simulink model "HipMotor"  (R2016a)
settings: Solver=VariableStepAuto  StartTime=0.0  StopTime=10.0  RelTol=1e-3
settings Model: Creator=MyPC  LastModifiedBy=MyPC

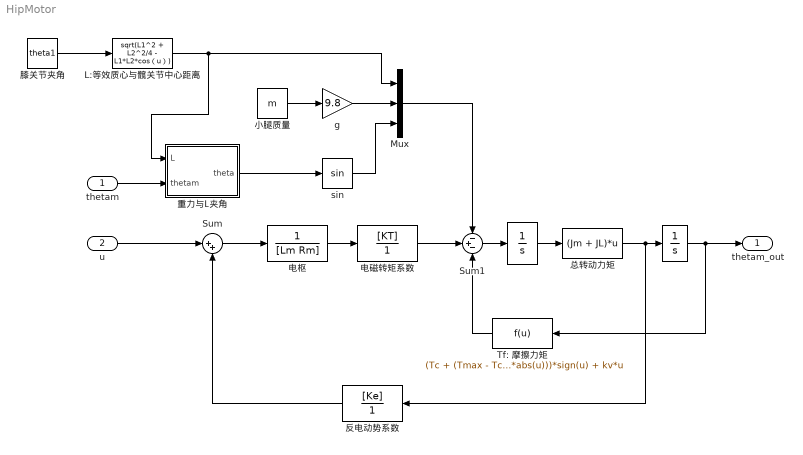
== system HipMotor ==
  thetam : Inport
  u : Inport  Port=2
  " " : TransferFcn  Denominator=[1 0]
  " " : TransferFcn  Denominator=[1 0]
  L:等效质心与髋关节中心距离 : Fcn  Expr=sqrt(L1^2 + L2^2/4 - L1*L2*cos（u）)  mask{L2=0.3, L1=0.3}
  Mux : Mux  Inputs=3
  Sum : Sum  Inputs=|++
  Sum1 : Sum  Inputs=-+-
  Tf: 摩擦力矩 : Fcn  Expr=(Tc + (Tmax - Tc)*exp(-v*abs(u)))*sign(u) + kv*u  mask{Tc=0.05, Tmax=0.06, v=0.01, kv=0.02}
  g : Gain  Gain=9.8
  sin : Trigonometry
  反电动势系数 : TransferFcn  Numerator=[Ke]  Denominator=[1]  mask{Ke=0.444}
  小腿质量 : Constant  Value=m  mask{m=5}
  总转动力矩 : Fcn  Expr=(Jm + JL)*u  mask{Jm=1.39e-4, JL=0.2}
  电枢 : TransferFcn  Denominator=[Lm Rm]  mask{Lm=2.34, Rm=5.48}
  电磁转矩系数 : TransferFcn  Numerator=[KT]  Denominator=[1]  mask{KT=0.443}
  膝关节夹角 : Constant  Value=theta1  mask{theta1=1.57}
  重力与L夹角 : MATLAB Function  TreatAsAtomicUnit=on  mask{L1=0.3, L2=0.3}
  thetam_out : Outport
  wires:
  u/1 -> Sum/1
  Sum/1 -> 电枢/1
  电枢/1 -> 电磁转矩系数/1
  电磁转矩系数/1 -> Sum1/2
  Sum1/1 -> " "/1
  Mux/1 -> Sum1/1
  小腿质量/1 -> g/1
  " "/1 -> 总转动力矩/1
  反电动势系数/1 -> Sum/2
  " "/1 -> thetam_out/1, Tf: 摩擦力矩/1
  sin/1 -> Mux/3
  g/1 -> Mux/2
  膝关节夹角/1 -> L:等效质心与髋关节中心距离/1
  L:等效质心与髋关节中心距离/1 -> 重力与L夹角/1(L), Mux/1
  Tf: 摩擦力矩/1 -> Sum1/3
  总转动力矩/1 -> 反电动势系数/1, " "/1
  重力与L夹角/1(theta) -> sin/1
  thetam/1 -> 重力与L夹角/2(thetam)

== matlab function HipMotor/重力与L夹角 ==
  data: L input; thetam input; theta output
function theta = fcn(L, thetam)

theta = pi - thetam - acos((L^2 + L1^2 - L2^2)/(2*L1*L));
